simulink model "sds1104receiver"  (R2023a)
settings: Solver=VariableStepAuto  StartTime=0.0  StopTime=inf  RelTol=1e-3
libraries: dspfdesign x32, simulink x1
settings Model: Creator=User  LastModifiedBy=User

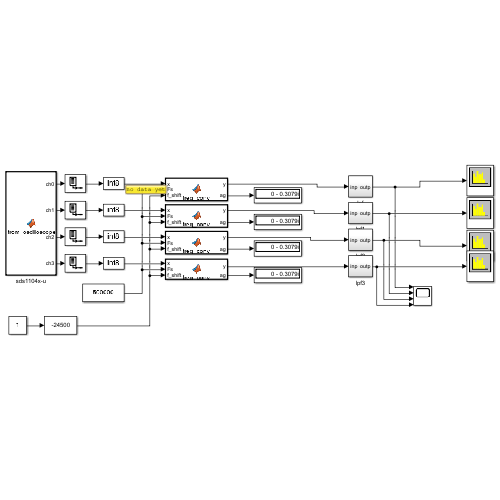
[thumbnail: Simulink's stored preview of the top-level diagram]
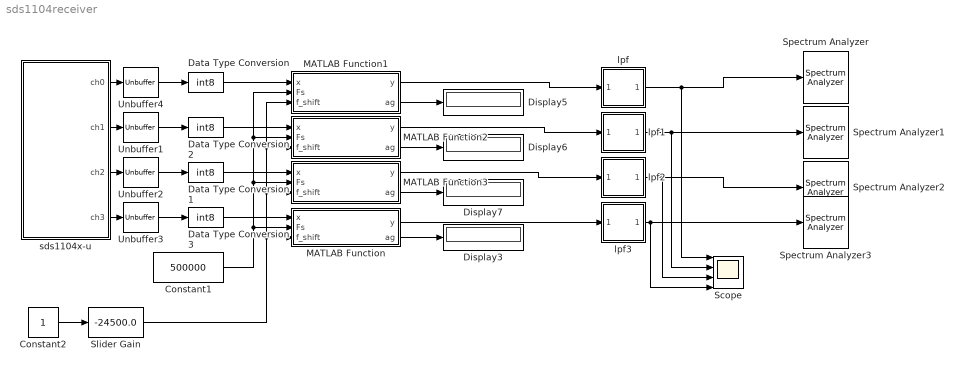
== system sds1104receiver ==
  Constant1 : Constant  Value=500000
  Constant2 : Constant
  Data Type Conversion{,1..3} (4 alike) : DataTypeConversion  OutDataTypeStr=int8  SaturateOnIntegerOverflow=off  RndMeth=Floor
  Display{3,5..7} (4 alike) : Display
  MATLAB Function : MATLAB Function  TreatAsAtomicUnit=on
  MATLAB Function1 : MATLAB Function  TreatAsAtomicUnit=on
  MATLAB Function2 : MATLAB Function  TreatAsAtomicUnit=on
  MATLAB Function3 : MATLAB Function  TreatAsAtomicUnit=on
  Scope : Scope  NumInputPorts=4
  Slider Gain : simulink/Math Operations/Slider Gain  gain=-24500.0  low=-50000  high=0
  Spectrum Analyzer : SpectrumAnalyzer  WindowPosition=[1198.000000,818.000000,800.000000,500.000000,]  Visible=on  ScopeFrameLocation=window  Span=1953.1249999999998  StartFrequency=-976.5624999999999  StopFrequency=976.5624999999999  YLimits=[-232.1866876,20.57316134]  ColorLimits=[-80 20]  SelectedToolstripTab=spectrumAnalyzerToolstrip.spectrumTab
  Spectrum Analyzer1 : SpectrumAnalyzer  WindowPosition=[331.000000,269.000000,800.000000,500.000000,]  Visible=on  ScopeFrameLocation=window  Span=499999.99999999994  StartFrequency=-249999.99999999997  StopFrequency=249999.99999999997  YLimits=[-7.16877835,57.05409486]  ColorLimits=[-80 20]  SelectedToolstripTab=spectrumAnalyzerToolstrip.spectrumTab
  Spectrum Analyzer2 : SpectrumAnalyzer  WindowPosition=[384.000000,818.000000,800.000000,500.000000,]  Visible=on  ScopeFrameLocation=window  Span=499999.99999999994  StartFrequency=-249999.99999999997  StopFrequency=249999.99999999997  YLimits=[-8.44829834,53.6642644]  ColorLimits=[-80 20]  SelectedToolstripTab=spectrumAnalyzerToolstrip.spectrumTab
  Spectrum Analyzer3 : SpectrumAnalyzer  WindowPosition=[581.000000,67.000000,800.000000,500.000000,]  Visible=on  ScopeFrameLocation=window  Span=499999.99999999994  StartFrequency=-249999.99999999997  StopFrequency=249999.99999999997  YLimits=[11.339,46.6379]  ColorLimits=[-80 20]  SelectedToolstripTab=spectrumAnalyzerToolstrip.spectrumTab
  Unbuffer{1..4} (4 alike) : Unbuffer
  lpf : Subsystem
  lpf1 : Subsystem
  lpf2 : Subsystem
  lpf3 : Subsystem
  sds1104x-u : MATLAB Function  TreatAsAtomicUnit=on  SystemSampleTime=7000/500000
  wires:
  sds1104x-u/2(ch1) -> Unbuffer1/1
  sds1104x-u/3(ch2) -> Unbuffer2/1
  sds1104x-u/4(ch3) -> Unbuffer3/1
  Unbuffer1/1 -> Data Type Conversion2/1
  Unbuffer2/1 -> Data Type Conversion1/1
  Unbuffer3/1 -> Data Type Conversion3/1
  sds1104x-u/1(ch0) -> Unbuffer4/1
  Unbuffer4/1 -> Data Type Conversion/1
  Data Type Conversion3/1 -> MATLAB Function/1(x)
  Constant1/1 -> MATLAB Function3/2(Fs), MATLAB Function2/2(Fs), MATLAB Function1/2(Fs), MATLAB Function/2(Fs)
  Constant2/1 -> Slider Gain/1
  Slider Gain/1 -> MATLAB Function2/3(f_shift), MATLAB Function1/3(f_shift), MATLAB Function3/3(f_shift), MATLAB Function/3(f_shift)
  MATLAB Function/1(y) -> lpf3/1(inp)
  MATLAB Function/2(ag) -> Display3/1
  Data Type Conversion/1 -> MATLAB Function1/1(x)
  Data Type Conversion2/1 -> MATLAB Function2/1(x)
  Data Type Conversion1/1 -> MATLAB Function3/1(x)
  MATLAB Function3/2(ag) -> Display7/1
  MATLAB Function2/2(ag) -> Display6/1
  MATLAB Function1/2(ag) -> Display5/1
  MATLAB Function1/1(y) -> lpf/1(inp)
  MATLAB Function2/1(y) -> lpf1/1(inp)
  MATLAB Function3/1(y) -> lpf2/1(inp)
  lpf/1(outp) -> Scope/1, Spectrum Analyzer/1
  lpf1/1(outp) -> Scope/2, Spectrum Analyzer1/1
  lpf2/1(outp) -> Scope/3, Spectrum Analyzer2/1
  lpf3/1(outp) -> Scope/4, Spectrum Analyzer3/1

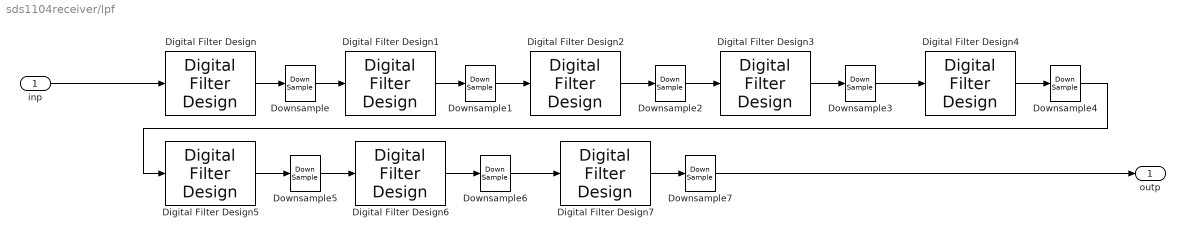
== system sds1104receiver/lpf ==
  inp : Inport
  Digital Filter Design{,1..7} (8 alike) : dspfdesign/Digital Filter Design  mwdsp_browser_bugfix_var=off
  Downsample{,1..7} (8 alike) : DownSample  RateOptions=Allow multirate processing
  outp : Outport
  wires:
  Downsample1/1 -> Digital Filter Design2/1
  Digital Filter Design5/1 -> Downsample5/1
  Digital Filter Design4/1 -> Downsample4/1
  Digital Filter Design7/1 -> Downsample7/1
  Downsample/1 -> Digital Filter Design1/1
  Downsample7/1 -> outp/1
  Downsample5/1 -> Digital Filter Design6/1
  Digital Filter Design/1 -> Downsample/1
  Digital Filter Design2/1 -> Downsample2/1
  Downsample3/1 -> Digital Filter Design4/1
  Downsample4/1 -> Digital Filter Design5/1
  Digital Filter Design3/1 -> Downsample3/1
  Downsample2/1 -> Digital Filter Design3/1
  Digital Filter Design6/1 -> Downsample6/1
  Digital Filter Design1/1 -> Downsample1/1
  Downsample6/1 -> Digital Filter Design7/1
  inp/1 -> Digital Filter Design/1

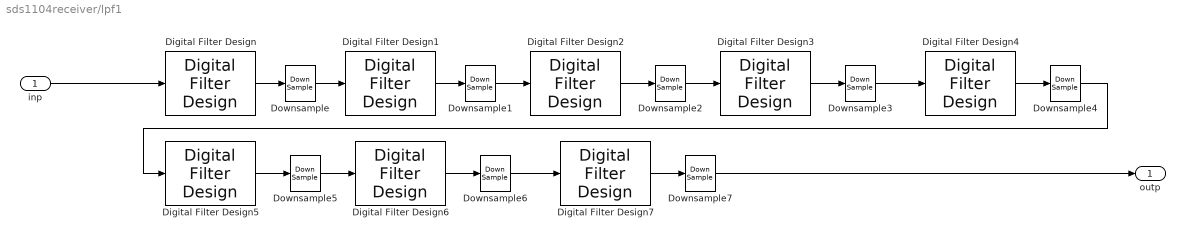
== system sds1104receiver/lpf1 ==
  inp : Inport
  Digital Filter Design{,1..7} (8 alike) : dspfdesign/Digital Filter Design  mwdsp_browser_bugfix_var=off
  Downsample{,1..7} (8 alike) : DownSample  RateOptions=Allow multirate processing
  outp : Outport
  wires:
  Downsample1/1 -> Digital Filter Design2/1
  Digital Filter Design5/1 -> Downsample5/1
  Digital Filter Design4/1 -> Downsample4/1
  Digital Filter Design7/1 -> Downsample7/1
  Downsample/1 -> Digital Filter Design1/1
  Downsample7/1 -> outp/1
  Downsample5/1 -> Digital Filter Design6/1
  Digital Filter Design/1 -> Downsample/1
  Digital Filter Design2/1 -> Downsample2/1
  Downsample3/1 -> Digital Filter Design4/1
  Downsample4/1 -> Digital Filter Design5/1
  Digital Filter Design3/1 -> Downsample3/1
  Downsample2/1 -> Digital Filter Design3/1
  Digital Filter Design6/1 -> Downsample6/1
  Digital Filter Design1/1 -> Downsample1/1
  Downsample6/1 -> Digital Filter Design7/1
  inp/1 -> Digital Filter Design/1

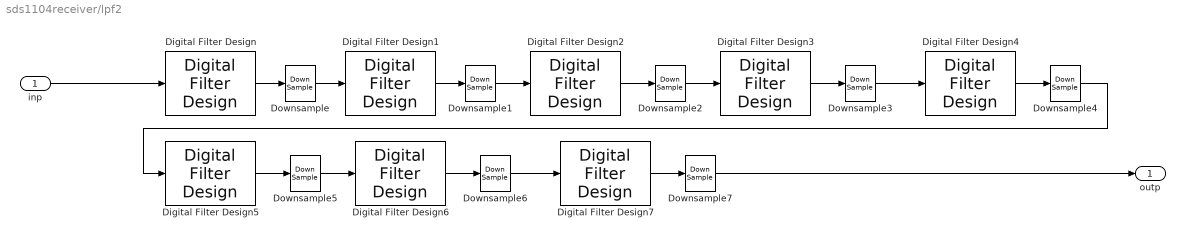
== system sds1104receiver/lpf2 ==
  inp : Inport
  Digital Filter Design{,1..7} (8 alike) : dspfdesign/Digital Filter Design  mwdsp_browser_bugfix_var=off
  Downsample{,1..7} (8 alike) : DownSample  RateOptions=Allow multirate processing
  outp : Outport
  wires:
  Downsample1/1 -> Digital Filter Design2/1
  Digital Filter Design5/1 -> Downsample5/1
  Digital Filter Design4/1 -> Downsample4/1
  Digital Filter Design7/1 -> Downsample7/1
  Downsample/1 -> Digital Filter Design1/1
  Downsample7/1 -> outp/1
  Downsample5/1 -> Digital Filter Design6/1
  Digital Filter Design/1 -> Downsample/1
  Digital Filter Design2/1 -> Downsample2/1
  Downsample3/1 -> Digital Filter Design4/1
  Downsample4/1 -> Digital Filter Design5/1
  Digital Filter Design3/1 -> Downsample3/1
  Downsample2/1 -> Digital Filter Design3/1
  Digital Filter Design6/1 -> Downsample6/1
  Digital Filter Design1/1 -> Downsample1/1
  Downsample6/1 -> Digital Filter Design7/1
  inp/1 -> Digital Filter Design/1

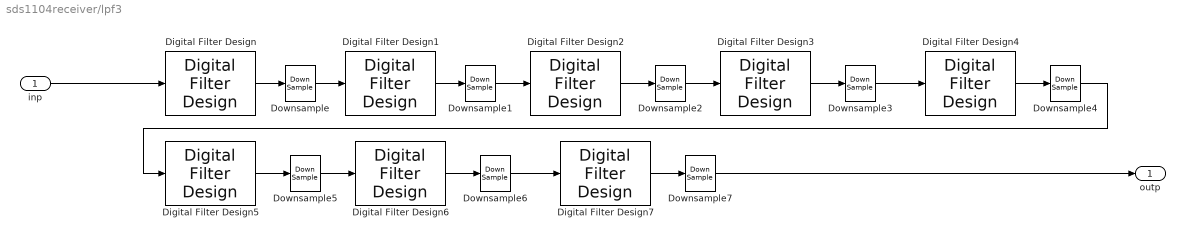
== system sds1104receiver/lpf3 ==
  inp : Inport
  Digital Filter Design{,1..7} (8 alike) : dspfdesign/Digital Filter Design  mwdsp_browser_bugfix_var=off
  Downsample{,1..7} (8 alike) : DownSample  RateOptions=Allow multirate processing
  outp : Outport
  wires:
  Downsample1/1 -> Digital Filter Design2/1
  Digital Filter Design5/1 -> Downsample5/1
  Digital Filter Design4/1 -> Downsample4/1
  Digital Filter Design7/1 -> Downsample7/1
  Downsample/1 -> Digital Filter Design1/1
  Downsample7/1 -> outp/1
  Downsample5/1 -> Digital Filter Design6/1
  Digital Filter Design/1 -> Downsample/1
  Digital Filter Design2/1 -> Downsample2/1
  Downsample3/1 -> Digital Filter Design4/1
  Downsample4/1 -> Digital Filter Design5/1
  Digital Filter Design3/1 -> Downsample3/1
  Downsample2/1 -> Digital Filter Design3/1
  Digital Filter Design6/1 -> Downsample6/1
  Digital Filter Design1/1 -> Downsample1/1
  Downsample6/1 -> Digital Filter Design7/1
  inp/1 -> Digital Filter Design/1

== matlab function sds1104receiver/MATLAB Function ==
  data: x input; y output; Fs input; f_shift input; ag output
function [y,ag]= freq_conv(x, Fs, f_shift)
% COMPLEX_DOWNCONVERTER Downconverts a real signal to complex baseband
%
% Inputs:
%   x       - real input signal (scalar or vector per time step)
%   Fs      - sampling rate (Hz)
%   f_shift - frequency to shift down (Hz)
%
% Output:
%   y       - complex baseband signal

% Persistent time vector to maintain phase continuity
persistent mx
ag = 1.0j*2*pi*double(f_shift)/double(Fs);
if isempty(mx)
    % Initialize time vector for the current frame
    mx = 1.0+0.0j;
else
    % Increment time for continuity
    mx = mx * exp(ag);
end

% Multiply real signal by complex exponential
y = double(x) * mx;
end

== matlab function sds1104receiver/sds1104x-u ==
  data: ch0 output; ch1 output; ch2 output; ch3 output
% this is for simulink matlab module
function [ch0,ch1,ch2,ch3] = read_file_from_oscilloscope_receiver()
    persistent buf
    N = 7000;
    if isempty(buf)
        buf = zeros(4*N,1,'uint8');
    end
    % Call helper function to get latest data
    buf = read_file_helper(N);
    ch0 = buf(1:N);
    ch1 = buf(N+1:2*N);
    ch2 = buf(2*N+1:3*N);
    ch3 = buf(3*N+1:4*N);
end

== matlab function sds1104receiver/MATLAB Function1 ==
  data: x input; y output; Fs input; f_shift input; ag output
function [y,ag]= freq_conv(x, Fs, f_shift)
% COMPLEX_DOWNCONVERTER Downconverts a real signal to complex baseband
%
% Inputs:
%   x       - real input signal (scalar or vector per time step)
%   Fs      - sampling rate (Hz)
%   f_shift - frequency to shift down (Hz)
%
% Output:
%   y       - complex baseband signal

% Persistent time vector to maintain phase continuity
persistent mx
ag = 1.0j*2*pi*double(f_shift)/double(Fs);
if isempty(mx)
    % Initialize time vector for the current frame
    mx = 1.0+0.0j;
else
    % Increment time for continuity
    mx = mx * exp(ag);
end

% Multiply real signal by complex exponential
y = double(x) * mx;
end

== matlab function sds1104receiver/MATLAB Function2 ==
  data: x input; y output; Fs input; f_shift input; ag output
function [y,ag]= freq_conv(x, Fs, f_shift)
% COMPLEX_DOWNCONVERTER Downconverts a real signal to complex baseband
%
% Inputs:
%   x       - real input signal (scalar or vector per time step)
%   Fs      - sampling rate (Hz)
%   f_shift - frequency to shift down (Hz)
%
% Output:
%   y       - complex baseband signal

% Persistent time vector to maintain phase continuity
persistent mx
ag = 1.0j*2*pi*double(f_shift)/double(Fs);
if isempty(mx)
    % Initialize time vector for the current frame
    mx = 1.0+0.0j;
else
    % Increment time for continuity
    mx = mx * exp(ag);
end

% Multiply real signal by complex exponential
y = double(x) * mx;
end

== matlab function sds1104receiver/MATLAB Function3 ==
  data: x input; y output; Fs input; f_shift input; ag output
function [y,ag]= freq_conv(x, Fs, f_shift)
% COMPLEX_DOWNCONVERTER Downconverts a real signal to complex baseband
%
% Inputs:
%   x       - real input signal (scalar or vector per time step)
%   Fs      - sampling rate (Hz)
%   f_shift - frequency to shift down (Hz)
%
% Output:
%   y       - complex baseband signal

% Persistent time vector to maintain phase continuity
persistent mx
ag = 1.0j*2*pi*double(f_shift)/double(Fs);
if isempty(mx)
    % Initialize time vector for the current frame
    mx = 1.0+0.0j;
else
    % Increment time for continuity
    mx = mx * exp(ag);
end

% Multiply real signal by complex exponential
y = double(x) * mx;
end
